simulink model "sim_demo_pendulum"  (R2021a)
settings: Solver=FixedStepAuto  StartTime=0.0  StopTime=0.5  FixedStep=1  RelTol=1e-3
settings Model: Creator=KBZeda  LastModifiedBy=KBZeda

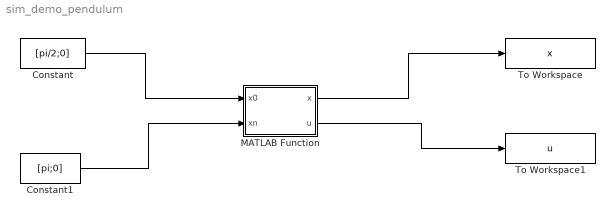
== system sim_demo_pendulum ==
  Constant : Constant  Value=[pi/2;0]
  Constant1 : Constant  Value=[pi;0]
  MATLAB Function : MATLAB Function  TreatAsAtomicUnit=on
  To Workspace : ToWorkspace  VariableName=x  SaveFormat=Timeseries  SampleTime=-1
  To Workspace1 : ToWorkspace  VariableName=u  SaveFormat=Timeseries  SampleTime=-1
  wires:
  Constant/1 -> MATLAB Function/1(x0)
  MATLAB Function/1(x) -> To Workspace/1
  Constant1/1 -> MATLAB Function/2(xn)
  MATLAB Function/2(u) -> To Workspace1/1

== matlab function sim_demo_pendulum/MATLAB Function ==
  data: x0 input; x output; xn input; u output
function [x, u] = fcn(x0, xn)


T       = 500;              % horizon
u0      = 10*randn(1,T);    % initial controls

%---------------------- user-adjustable parameters ------------------------
defaults = {'lims',           [],...            control limits
            'parallel',       true,...          use parallel line-search?
            'Alpha',          10.^linspace(0,-3,11),... backtracking coefficients
            'tolFun',         1e-7,...          reduction exit criterion
            'tolGrad',        1e-4,...          gradient exit criterion
            'maxIter',        500,...           maximum iterations            
            'lambda',         1,...             initial value for lambda
            'dlambda',        1,...             initial value for dlambda
            'lambdaFactor',   1.6,...           lambda scaling factor
            'lambdaMax',      1e10,...          lambda maximum value
            'lambdaMin',      1e-6,...          below this value lambda = 0
            'regType',        1,...             regularization type 1: q_uu+lambda*eye(); 2: V_xx+lambda*eye()
            'zMin',           0,...             minimal accepted reduction ratio
            'diffFn',         [],...            user-defined diff for sub-space optimization
            'plot',           1,...             0: no;  k>0: every k iters; k<0: every k iters, with derivs window
            'print',          2,...             0: no;  1: final; 2: iter; 3: iter, detailed
            'plotFn',         @(x)0,...         user-defined graphics callback
            'cost',           [],...            initial cost for pre-rolled trajectory            
            };

        
% --- initial sizes and controls
n   = size(x0, 1);          % dimension of state vector
m   = size(u0, 1);          % dimension of control vector
N   = size(u0, 2);          % number of state transitions
u   = u0;                   % initial control sequence

%Op = struct();
Op.lims = [-10000 10000];   % external force (N)
Op.plot = -1;               % plot the derivatives as well

%line_handle = line([0 0],[0 0],'color','b','linewidth',2);
% plotFn = @(x) set(line_handle,'Xdata',x(1,:),'Ydata',x(2,:));
% Op.plotFn = plotFn;


Op  = setOpts(defaults,Op);

verbosity = Op.print;

switch numel(Op.lims)
    case 0
    case 2*m
        Op.lims = sort(Op.lims,2);
    case 2
        Op.lims = ones(m,1)*sort(Op.lims(:))';
    case m
        Op.lims = Op.lims(:)*[-1 1];
    otherwise
        error('limits are of the wrong size')
end


lambda   = Op.lambda;
dlambda  = Op.dlambda;

% --- initialize trace data structure
trace = struct('iter',nan,'lambda',nan,'dlambda',nan,'cost',nan,...
        'alpha',nan,'grad_norm',nan,'improvement',nan,'reduc_ratio',nan,...
        'time_derivs',nan,'time_forward',nan,'time_backward',nan);
trace = repmat(trace,[min(Op.maxIter,1e6) 1]);
trace(1).iter = 1;
trace(1).lambda = lambda;
trace(1).dlambda = dlambda;


% --- initial trajectory
if size(x0,2) == 1
    diverge = true;
    for alpha = Op.Alpha
        x = x0;  %forward_pass(x0(:,1),alpha*u,[],[],[],1,Op.lims,[]);
        un = u;
        % simplistic divergence test
        if all(abs(x(:)) < 1e8)
            u = un;
            diverge = false;
            break
        end
    end
elseif size(x0,2) == N+1 % pre-rolled initial forward pass
    x        = x0;
    diverge  = false;
    if isempty(Op.cost)
        error('pre-rolled initial trajectory requires cost')
    else
        cost     = Op.cost;
    end
else
    error('pre-rolled initial trajectory must be of correct length')
end

trace(1).cost = sum(cost(:));


if diverge
    [Vx,Vxx, stop]  = deal(nan);
    L        = zeros(m,n,N);
    cost     = [];
    trace    = trace(1);
    if verbosity > 0
        fprintf('\nEXIT: Initial control sequence caused divergence\n');
    end
    return
end

% % constants, timers, counters
% flgChange   = 1;
% stop        = 0;
% dcost       = 0;
% z           = 0;
% expected    = 0;
% print_head  = 6; % print headings every print_head lines
% last_head   = print_head;
% t_start     = tic;
% if verbosity > 0
%     fprintf('\n=========== begin iLQG ===========\n');
% end
% 
% for iter = 1:Op.maxIter
%     if stop
%         break;
%     end
%     trace(iter).iter = iter;    
%     
%     %====== STEP 1: differentiate dynamics and cost along new trajectory
%     if flgChange
%         t_diff = tic;
%         [~,~,fx,fu,fxx,fxu,fuu,cx,cu,cxx,cxu,cuu]   = pendulum_dyn_cst(x, [u nan(m,1)], 1:N+1);
%         trace(iter).time_derivs = toc(t_diff);
%         flgChange   = 0;
%     end
%     
%     %====== STEP 2: backward pass, compute optimal control law and cost-to-go
%     backPassDone   = 0;
%     while ~backPassDone
%         
%         t_back   = tic;
%         [diverge, Vx, Vxx, l, L, dV] = back_pass(cx,cu,cxx,cxu,cuu,fx,fu,fxx,fxu,fuu,lambda,Op.regType,Op.lims,u);
%         trace(iter).time_backward = toc(t_back);
%         trace(iter).k = l;
%         trace(iter).K = L;
%         
%         if diverge
%             if verbosity > 2
%                 fprintf('Cholesky failed at timestep %d.\n',diverge);
%             end
%             dlambda   = max(dlambda * Op.lambdaFactor, Op.lambdaFactor);
%             lambda    = max(lambda * dlambda, Op.lambdaMin);
%             if lambda > Op.lambdaMax
%                 break;
%             end
%             continue
%         end
%         backPassDone      = 1;
%     end
% 
%     % check for termination due to small gradient
%     g_norm         = mean(max(abs(l) ./ (abs(u)+1),[],1));
%     trace(iter).grad_norm = g_norm;
%     if g_norm < Op.tolGrad && lambda < 1e-5
%         dlambda   = min(dlambda / Op.lambdaFactor, 1/Op.lambdaFactor);
%         lambda    = lambda * dlambda * (lambda > Op.lambdaMin);
%         if verbosity > 0
%             fprintf('\nSUCCESS: gradient norm < tolGrad\n');
%         end
%         break;
%     end
%     
%     %====== STEP 3: line-search to find new control sequence, trajectory, cost
%     fwdPassDone  = 0;
%     if backPassDone
%         t_fwd = tic;
%         if Op.parallel  % parallel line-search
%             [xnew,unew,costnew] = forward_pass(x0 ,u, L, x(:,1:N), l, Op.Alpha,Op.lims,Op.diffFn);
%             Dcost               = sum(cost(:)) - sum(costnew,2);
%             [dcost, w]          = max(Dcost);
%             alpha               = Op.Alpha(w);
%             expected            = -alpha*(dV(1) + alpha*dV(2));
%             if expected > 0
%                 z = dcost/expected;
%             else
%                 z = sign(dcost);
%                 warning('non-positive expected reduction: should not occur');
%             end
%             if (z > Op.zMin)
%                 fwdPassDone = 1;
%                 costnew     = costnew(:,:,w);
%                 xnew        = xnew(:,:,w);
%                 unew        = unew(:,:,w);
%             end
%         else            % serial backtracking line-search
%             for alpha = Op.Alpha
%                 [xnew,unew,costnew]   = forward_pass(x0 ,u+l*alpha, L, x(:,1:N),[],1,Op.lims,Op.diffFn);
%                 dcost    = sum(cost(:)) - sum(costnew(:));
%                 expected = -alpha*(dV(1) + alpha*dV(2));
%                 if expected > 0
%                     z = dcost/expected;
%                 else
%                     z = sign(dcost);
%                     warning('non-positive expected reduction: should not occur');
%                 end
%                 if (z > Op.zMin)
%                     fwdPassDone = 1;
%                     break;
%                 end
%             end
%         end
%         if ~fwdPassDone
%             alpha = nan; % signals failure of forward pass
%         end
%         trace(iter).time_forward = toc(t_fwd);
%     end
%     
%     %====== STEP 4: accept step (or not), draw graphics, print status
%     
%     % print headings
%     if verbosity > 1 && last_head == print_head
%         last_head = 0;
%         fprintf('%-12s','iteration','cost','reduction','expected','gradient','log10(lambda)')
%         fprintf('\n');
%     end
%     
%     if fwdPassDone
%         
%         % print status
%         if verbosity > 1
%             fprintf('%-12d%-12.6g%-12.3g%-12.3g%-12.3g%-12.1f\n', ...
%                 iter, sum(cost(:)), dcost, expected, g_norm, log10(lambda));
%             last_head = last_head+1;
%         end
%         
%         % decrease lambda
%         dlambda   = min(dlambda / Op.lambdaFactor, 1/Op.lambdaFactor);
%         lambda    = lambda * dlambda * (lambda > Op.lambdaMin);
%         
%         % accept changes
%         u              = unew;
%         x              = xnew;
%         cost           = costnew;
%         flgChange      = 1;
%         Op.plotFn(x);
%         
%         % terminate ?
%         if dcost < Op.tolFun
%             if verbosity > 0
%                 fprintf('\nSUCCESS: cost change < tolFun\n');
%             end
%             break;
%         end
%         
%     else % no cost improvement
%         % increase lambda
%         dlambda  = max(dlambda * Op.lambdaFactor, Op.lambdaFactor);
%         lambda   = max(lambda * dlambda, Op.lambdaMin);
%         
%         % print status
%         if verbosity > 1
%             fprintf('%-12d%-12s%-12.3g%-12.3g%-12.3g%-12.1f\n', ...
%                 iter,'NO STEP', dcost, expected, g_norm, log10(lambda));           
%             last_head = last_head+1;
%         end     
%         
%         % terminate ?
%         if lambda > Op.lambdaMax
%             if verbosity > 0
%                 fprintf('\nEXIT: lambda > lambdaMax\n');
%             end
%             break;
%         end
%     end
%     % update trace
%     trace(iter).lambda      = lambda;
%     trace(iter).dlambda     = dlambda;
%     trace(iter).alpha       = alpha;
%     trace(iter).improvement = dcost;
%     trace(iter).cost        = sum(cost(:));
%     trace(iter).reduc_ratio = z;
%     %stop = graphics(Op.plot,x,u,cost,L,Vx,Vxx,fx,fxx,fu,fuu,trace(1:iter),0);
% end
% 
% 
% 
% % save lambda/dlambda
% trace(iter).lambda      = lambda;
% trace(iter).dlambda     = dlambda;
% 
% if stop && (verbosity > 0)
%         fprintf('\nEXIT: Terminated by user\n');
% end
% 
% if iter == Op.maxIter
%     if verbosity > 0
%         fprintf('\nEXIT: Maximum iterations reached.\n');
%     end
% end
% 
% 
% if ~isempty(iter)
%     diff_t = [trace(1:iter).time_derivs];
%     diff_t = sum(diff_t(~isnan(diff_t)));
%     back_t = [trace(1:iter).time_backward];
%     back_t = sum(back_t(~isnan(back_t)));
%     fwd_t = [trace(1:iter).time_forward];
%     fwd_t = sum(fwd_t(~isnan(fwd_t)));
%     total_t = toc(t_start);
%     if verbosity > 0
%         fprintf(['\n'...
%             'iterations:   %-3d\n'...
%             'final cost:   %-12.7g\n' ...
%             'final grad:   %-12.7g\n' ...
%             'final lambda: %-12.7e\n' ...
%             'time / iter:  %-5.0f ms\n'...
%             'total time:   %-5.2f seconds, of which\n'...
%             '  derivs:     %-4.1f%%\n'...
%             '  back pass:  %-4.1f%%\n'...
%             '  fwd pass:   %-4.1f%%\n'...
%             '  other:      %-4.1f%% (graphics etc.)\n'...
%             '=========== end iLQG ===========\n'],...
%             iter,sum(cost(:)),g_norm,lambda,1e3*total_t/iter,total_t,...
%             [diff_t, back_t, fwd_t, (total_t-diff_t-back_t-fwd_t)]*100/total_t);
%     end
%     trace    = trace(~isnan([trace.iter]));
% %     timing   = [diff_t back_t fwd_t total_t-diff_t-back_t-fwd_t];
%     %graphics(Op.plot,x,u,cost,L,Vx,Vxx,fx,fxx,fu,fuu,trace,2); % draw legend
% else
%     error('Failure: no iterations completed, something is wrong.')
% end  
end
